simulink model "model0_RealizeODE"  (R2020a)
settings: Solver=FixedStepAuto  StartTime=0.0  StopTime=10  FixedStep=1e-3  RelTol=1e-3
InitFcn:
  | clear;clc
  | b = [ 0 1 2 16];
  | a = [ 9 28 30 16];
  | 
  | num = b;
  | den = [1 a];
StopFcn:
  | figure('name','result','windowstyle','normal')
  | plot(t,y1,'LineWidth',2,'Color','#2d85f0')
  | hold on
  | grid on
  | plot(t,y2,'LineWidth',2,'Color','#f4433c','Linestyle','--')
  | plot(t,y3,'LineWidth',2,'Color','#ffbc32','Linestyle',':')
  | xlabel('Time (s)')
  | ylabel('Response')
  | legend('Transfer Function','Control Canonical',...
  |      'Observer Canonical','Location','best')
settings Model: Creator=XiaoCY  LastModifiedBy=XiaoCY
settings DataIOCC: ReturnWorkspaceOutputs=off

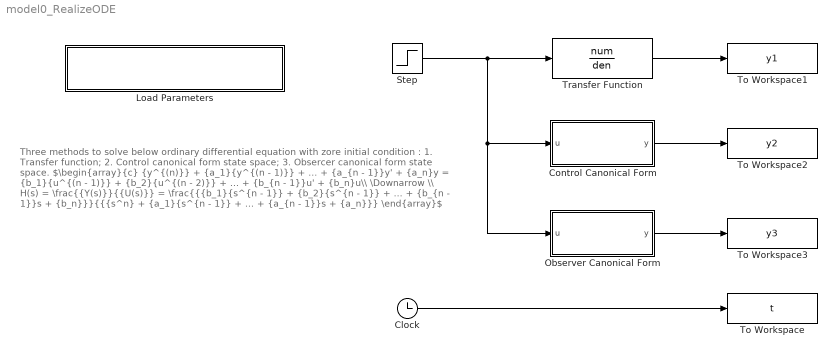
== system model0_RealizeODE ==
  note: Three methods to solve below ordinary differential equation with zore initial condition :
      | 1. Transfer function;
      | 2. Control canonical form state space;
      | 3. Obsercer canonical form state space.
      |
      | $\begin{array}{c} {y^{(n)}} + {a_1}{y^{(n - 1)}} + ... + {a_{n - 1}}y' + {a_n}y = {b_1}{u^{(n - 1)}} + {b_2}{u^{(n - 2)}} + ... + {b_{n - 1}}u' + {b_n}u\\ \Downarrow \\ H(s) = \frac{{Y(s)}}{{U(s)}} = \frac{{{b_1}{s^{n - 1}} + {b_2}{s^{n - 1}} + ... + {b_{n - 1}}s + {b_n}}}{{{s^n} + {a_1}{s^{n - 1}} + ... + {a_{n - 1}}s + {a_n}}} \end{array}$
  Clock : Clock
  Control Canonical Form : Subsystem
  Load Parameters : Subsystem
      settings: OpenFcn=sim('model0_RealizeODE.slx')
      mask Display: disp('Double click to run and view result.')
  Observer Canonical Form : Subsystem
  Step : Step  Time=0  SampleTime=0
  To Workspace : ToWorkspace  VariableName=t  SampleTime=-1
  To Workspace1 : ToWorkspace  VariableName=y1  SampleTime=-1
  To Workspace2 : ToWorkspace  VariableName=y2  SampleTime=-1
  To Workspace3 : ToWorkspace  VariableName=y3  SampleTime=-1
  Transfer Function : TransferFcn  Numerator=num  Denominator=den
  wires:
  Step/1 -> Observer Canonical Form/1(u), Control Canonical Form/1(u), Transfer Function/1
  Clock/1 -> To Workspace/1
  Transfer Function/1 -> To Workspace1/1
  Control Canonical Form/1(y) -> To Workspace2/1
  Observer Canonical Form/1(y) -> To Workspace3/1

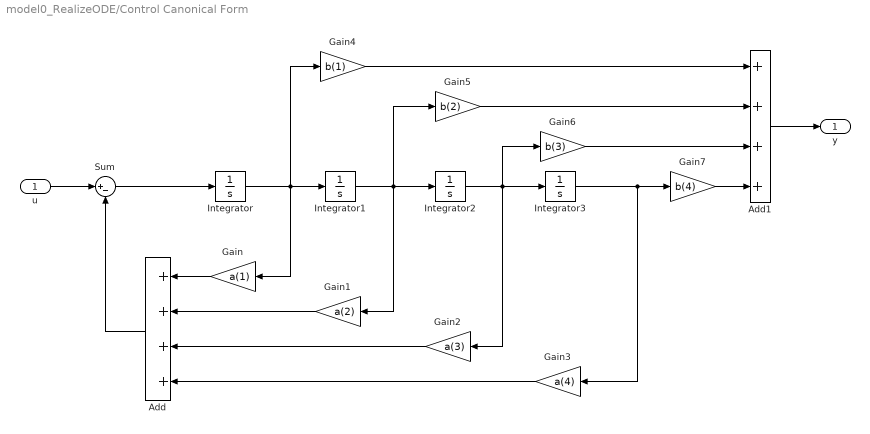
== system model0_RealizeODE/Control Canonical Form ==
  u : Inport
  Add : Sum  Inputs=++++
  Add1 : Sum  Inputs=++++
  Gain : Gain  Gain=a(1)
  Gain1 : Gain  Gain=a(2)
  Gain2 : Gain  Gain=a(3)
  Gain3 : Gain  Gain=a(4)
  Gain4 : Gain  Gain=b(1)
  Gain5 : Gain  Gain=b(2)
  Gain6 : Gain  Gain=b(3)
  Gain7 : Gain  Gain=b(4)
  Integrator{,1..3} (4 alike) : Integrator
  Sum : Sum  Inputs=|+-
  y : Outport
  wires:
  Integrator/1 -> Gain4/1, Gain/1, Integrator1/1
  Integrator1/1 -> Gain5/1, Gain1/1, Integrator2/1
  Integrator2/1 -> Gain6/1, Gain2/1, Integrator3/1
  Sum/1 -> Integrator/1
  u/1 -> Sum/1
  Add/1 -> Sum/2
  Gain/1 -> Add/1
  Gain1/1 -> Add/2
  Gain2/1 -> Add/3
  Integrator3/1 -> Gain7/1, Gain3/1
  Gain3/1 -> Add/4
  Add1/1 -> y/1
  Gain4/1 -> Add1/1
  Gain5/1 -> Add1/2
  Gain6/1 -> Add1/3
  Gain7/1 -> Add1/4

== system model0_RealizeODE/Load Parameters ==

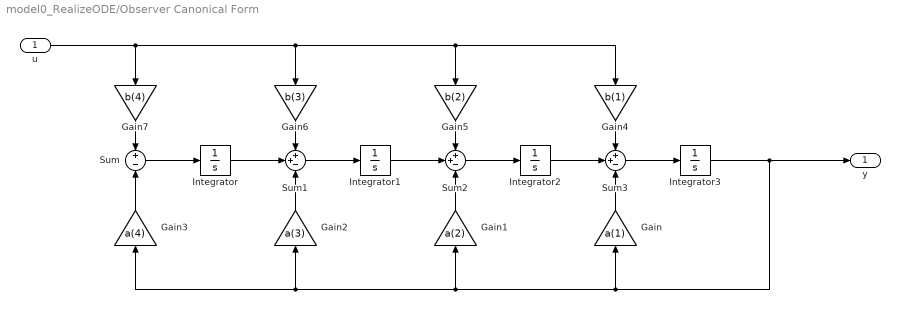
== system model0_RealizeODE/Observer Canonical Form ==
  u : Inport
  Gain : Gain  Gain=a(1)
  Gain1 : Gain  Gain=a(2)
  Gain2 : Gain  Gain=a(3)
  Gain3 : Gain  Gain=a(4)
  Gain4 : Gain  Gain=b(1)
  Gain5 : Gain  Gain=b(2)
  Gain6 : Gain  Gain=b(3)
  Gain7 : Gain  Gain=b(4)
  Integrator{,1..3} (4 alike) : Integrator
  Sum : Sum  Inputs=+|-
  Sum1 : Sum  Inputs=++-
  Sum2 : Sum  Inputs=++-
  Sum3 : Sum  Inputs=++-
  y : Outport
  wires:
  Sum/1 -> Integrator/1
  Integrator/1 -> Sum1/2
  Sum1/1 -> Integrator1/1
  Integrator1/1 -> Sum2/2
  Sum2/1 -> Integrator2/1
  Integrator2/1 -> Sum3/2
  Sum3/1 -> Integrator3/1
  Integrator3/1 -> Gain1/1, Gain2/1, Gain3/1, Gain/1, y/1
  Gain/1 -> Sum3/3
  Gain1/1 -> Sum2/3
  Gain3/1 -> Sum/2
  Gain2/1 -> Sum1/3
  u/1 -> Gain6/1, Gain5/1, Gain4/1, Gain7/1
  Gain4/1 -> Sum3/1
  Gain5/1 -> Sum2/1
  Gain6/1 -> Sum1/1
  Gain7/1 -> Sum/1
